simulink model "qw_laser_response"  (R2026a)
settings: Solver=ode4  StopTime=100e-9  FixedStep=1e-12
values from neighbouring files (symbols this model uses):
  eps_val = eps_val_cm3 * 1e-6    (= 3.4e-29)    [rate_equations_init.m]
  G_I = 1 / (q * Vact)    [rate_equations_init.m]
  G_N_decay = 1 / tau_n    [rate_equations_init.m]
  G_Ne = Ne / tau_n    [rate_equations_init.m]
  G_Pf = (Vact * eta * h * c) / (Gamma * tau_p * lambda0)    [rate_equations_init.m]
  G_S_decay = 1 / tau_p    [rate_equations_init.m]
Description:
  | Author: Puspendu Rana
  | Project: QW Laser Simulation
  | Date: April 2026
settings Model: Creator=Puspendu Rana  LastModifiedBy=HP

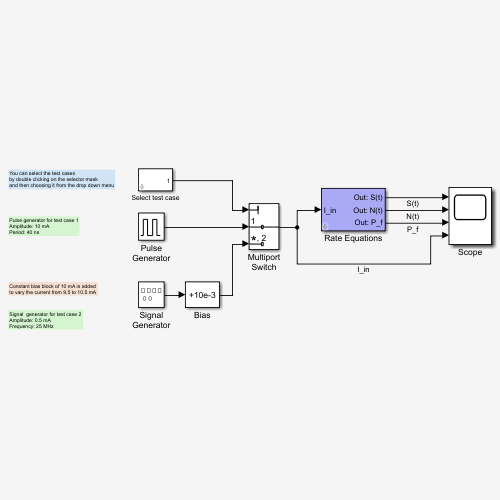
[thumbnail: Simulink's stored preview of the top-level diagram]
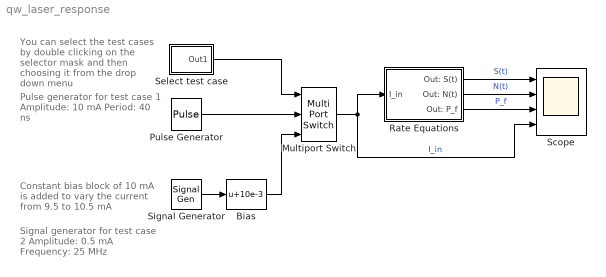
== system qw_laser_response ==
  note: Signal generator for test case 2
      | Amplitude: 0.5 mA
      | Frequency: 25 MHz
  note: Constant bias block of 10 mA is added
      | to vary the current from 9.5 to 10.5 mA
  note: Pulse generator for test case 1
      | Amplitude: 10 mA
      | Period: 40 ns
  note: You can select the test cases
      | by double clicking on the selector mask
      | and then choosing it from the drop down menu
  Bias : Bias  Bias=10e-3  SaturateOnIntegerOverflow=off
  Multiport Switch : MultiPortSwitch  Inputs=2  SaturateOnIntegerOverflow=off  InputSameDT=off
  Pulse Generator : DiscretePulseGenerator  PulseType=Time based  Amplitude=10e-3  Period=40e-9  PulseWidth=50
  Rate Equations : Subsystem  mask(Rate Equation){lambda0=1.502e-4, Vact=9e-11, Gamma=0.44, tau_n=3000, tau_p=1, g0=3e-6, beta=4e-4, N0=1.2e18, Ne=5.41e10, eta=0.1}
      mask prompts: lambda0 "Lasing wavelength (cm)"; Vact "Active region volume (cm³)"; Gamma "Optical Confinement factor"; tau_n "Carrier lifetime (ps)"; tau_p "Photon lifetime (ps)"; g0 "Gain coefficient (cm³/s)"; beta "Spontaneous emission coupling factor"; N0 "Optical transparency density (1/cm³)"; Ne "Equilibrium carrier density (1/cm³)"; eta "Differential quantum efficiency per facet"
      mask help: This subsystem implements a large-signal, time-domain simulation of a Quantum-Well LASER diode. Unlike small-signal frequency transfer functions, this block directly integrates the coupled non-linear rate equations for carrier density N(t) and photon density S(t) to accurately capture complex transient behaviors.
      mask DialogControl Container4 Prompt: Cavity Dimensions and Optical Confinement
      mask DialogControl Container5 Prompt: Carrier Dynamics and Gain
      mask DialogControl Container6 Prompt: Operating Densities and Efficiency
  Scope : Scope  NumInputPorts=4
      settings: ActiveDisplayString=4  Title=Injected Drive Current  ActiveDisplayYMinimum=0.009375  ActiveDisplayYMaximum=0.010625  YLabel=Drive Current, I(t) (A)
  Select test case : Subsystem  mask{test_selector=Test Case 2: 9.5 to 10.5 mA}
      mask prompts: test_selector "Select Test Cases:"
      mask TypeOptions test_selector: Test Case 1: 0 to 10 mA | Test Case 2: 9.5 to 10.5 mA
  Signal Generator : SignalGenerator  WaveForm=square  Amplitude=0.5e-3  Frequency=25e6
  wires:
  Rate Equations/1(Out: S(t)) -> Scope/1  "S(t)"
  Rate Equations/2(Out: N(t)) -> Scope/2  "N(t)"
  Rate Equations/3(Out: P_f) -> Scope/3  "P_f"
  Multiport Switch/1 -> Scope/4, Rate Equations/1(I_in)  "I_in"
  Select test case/1(Out1) -> Multiport Switch/1
  Signal Generator/1 -> Bias/1
  Bias/1 -> Multiport Switch/3
  Pulse Generator/1 -> Multiport Switch/2

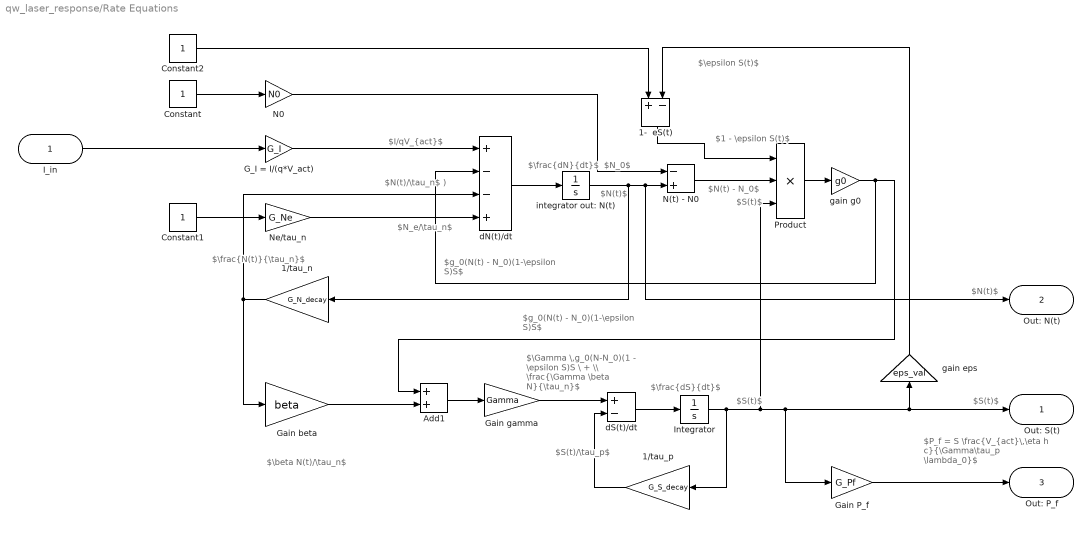
== system qw_laser_response/Rate Equations ==
  note: $S(t)$
  note: $P_f = S \frac{V_{act}\,\eta h c}{\Gamma\tau_p \lambda_0}$
  note: $\epsilon S(t)$
  note: $S(t)$
  note: $\frac{dS}{dt}$
  note: $\Gamma \,g_0(N-N_0)(1 - \epsilon S)S \ + \\ \frac{\Gamma \beta N}{\tau_n}$
  note: $S(t)/\tau_p$
  note: $\beta N(t)/\tau_n$
  note: $1 - \epsilon S(t)$
  note: $N(t) - N_0$
  note: $S(t)$
  note: $N_0$
  note: $N(t)$
  note: $\frac{dN}{dt}$
  note: $N_e/\tau_n$
  note: $I/qV_{act}$
  note: $\frac{N(t)}{\tau_n}$
  note: $g_0(N(t) - N_0)(1-\epsilon S)S$
  note: $N(t)/\tau_n$ )
  note: $g_0(N(t) - N_0)(1-\epsilon S)S$
  note: $N(t)$
  I_in : Inport
  1-  eS(t) : Sum  Inputs=+-
  1/tau_n : Gain  Gain=G_N_decay
  1/tau_p : Gain  Gain=G_S_decay
  Add1 : Sum
  Constant : Constant
  Constant1 : Constant
  Constant2 : Constant
  G_I = I/(q*V_act) : Gain  Gain=G_I
  Gain P_f : Gain  Gain=G_Pf
  Gain beta : Gain  Gain=beta
  Gain gamma : Gain  Gain=Gamma
  Integrator : Integrator
  N(t) - N0 : Sum  Inputs=-+
  N0 : Gain  Gain=N0
  Ne/tau_n : Gain  Gain=G_Ne
  Product : Product  Inputs=3
  dN(t)/dt : Sum  Inputs=+--+
  dS(t)/dt : Sum  Inputs=+-
  gain eps : Gain  Gain=eps_val
  gain g0 : Gain  Gain=g0
  integrator out: N(t) : Integrator
  Out: S(t) : Outport
  Out: N(t) : Outport  Port=2
  Out: P_f : Outport  Port=3
  wires:
  I_in/1 -> G_I = I/(q*V_act)/1
  Constant/1 -> N0/1
  G_I = I/(q*V_act)/1 -> dN(t)/dt/1
  dN(t)/dt/1 -> integrator out: N(t)/1
  integrator out: N(t)/1 -> 1/tau_n/1, Out: N(t)/1, N(t) - N0/2
  N0/1 -> N(t) - N0/1
  Constant1/1 -> Ne/tau_n/1
  Ne/tau_n/1 -> dN(t)/dt/4
  1/tau_n/1 -> Gain beta/1, dN(t)/dt/3
  Gain beta/1 -> Add1/2
  Add1/1 -> Gain gamma/1
  Gain gamma/1 -> dS(t)/dt/1
  dS(t)/dt/1 -> Integrator/1
  Integrator/1 -> 1/tau_p/1, Out: S(t)/1, gain eps/1, Gain P_f/1, Product/3
  1/tau_p/1 -> dS(t)/dt/2
  Constant2/1 -> 1-  eS(t)/1
  gain eps/1 -> 1-  eS(t)/2
  1-  eS(t)/1 -> Product/1
  N(t) - N0/1 -> Product/2
  Product/1 -> gain g0/1
  gain g0/1 -> dN(t)/dt/2, Add1/1
  Gain P_f/1 -> Out: P_f/1

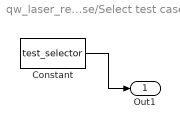
== system qw_laser_response/Select test case ==
  Constant : Constant  Value=test_selector
  Out1 : Outport
  wires:
  Constant/1 -> Out1/1
